simulink model "SpeedLoop"  (R2023b)
settings: Solver=FixedStepAuto  StartTime=0.0  StopTime=10.0  FixedStep=0.0001  RelTol=1e-3
values from neighbouring files (symbols this model uses):
  curr_ki = 2.3    [Speedloop.sldd]
  curr_kp = 0.0008    [Speedloop.sldd]
  Pn = 4.0    [Speedloop.sldd]
  spd_ki = 0.021    [Speedloop.sldd]
  spd_kp = 0.013    [Speedloop.sldd]
  Udc = 24.0    [Speedloop.sldd]
libraries: slpidlib x3, mcbplantlib x1, autolibpmsmexterior x1, simulink x1
settings Model: DataDictionary=Speedloop.sldd  Creator=00033411  LastModifiedBy=00033411
settings OptimizationCC: DefaultParameterBehavior=Inlined  UseDivisionForNetSlopeComputation=on  GainParamInheritBuiltInType=on  UseFloatMulNetSlope=on  InlineInvariantSignals=on  PassReuseOutputArgsAs=Individual arguments  ZeroExternalMemoryAtStartup=off  ZeroInternalMemoryAtStartup=off  NoFixptDivByZeroProtection=on  EfficientFloat2IntCast=on  LifeSpan=1  OptimizeBlockOrder=speed  DifferentSizesBufferReuse=on  EfficientTunableParamExpr=on
settings DebuggingCC: ParameterPrecisionLossMsg=none  ParameterTunabilityLossMsg=error
settings HardwareCC: ProdBitPerPointer=32  ProdBitPerSizeT=32  ProdBitPerPtrDiffT=32  ProdLargestAtomicInteger=Long  ProdLargestAtomicFloat=Double  ProdWordSize=32  ProdLongLongMode=on  ProdHWDeviceType=ARM Compatible->ARM Cortex-M
settings SFSimCC: MATLABDynamicMemAlloc=off
settings RTWCC: Description=Embedded Coder  SystemTargetFile=ert.tlc  TemplateMakefile=ert_default_tmf  GenerateReport=on  LaunchReport=on
settings CodeAppCC: ForceParamTrailComments=on  IgnoreCustomStorageClasses=off  OperatorAnnotations=on  SimulinkDataObjDesc=on  SFDataObjDesc=on  CustomSymbolStrGlobalVar=rt$N$M  CustomSymbolStrType=$N$M  CustomSymbolStrFcn=$N$M$F  CustomSymbolStrMacro=$N$M  InsertBlockDesc=on
settings ERTTargetCC: TargetLangStandard=C99 (ISO)  CodeReplacementLibrary=ARM Cortex-M  GenerateSampleERTMain=on  IncludeMdlTerminateFcn=off  CombineSignalStateStructs=on  SupportComplex=off  SupportNonInlinedSFcns=on  InlinedParameterPlacement=NonHierarchical  ERTCustomFileTemplate=example_file_process.tlc  ERTFilePackagingFormat=CompactWithDataFile

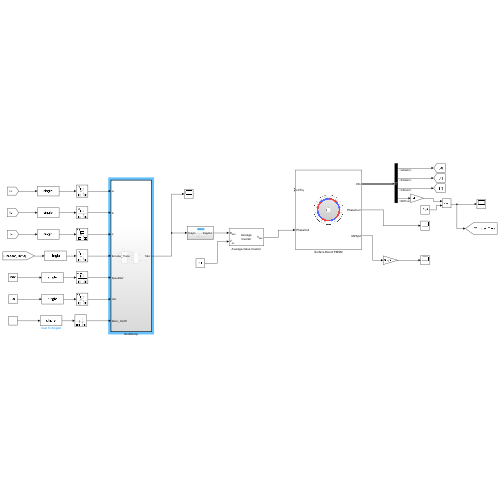
[thumbnail: Simulink's stored preview of the top-level diagram]
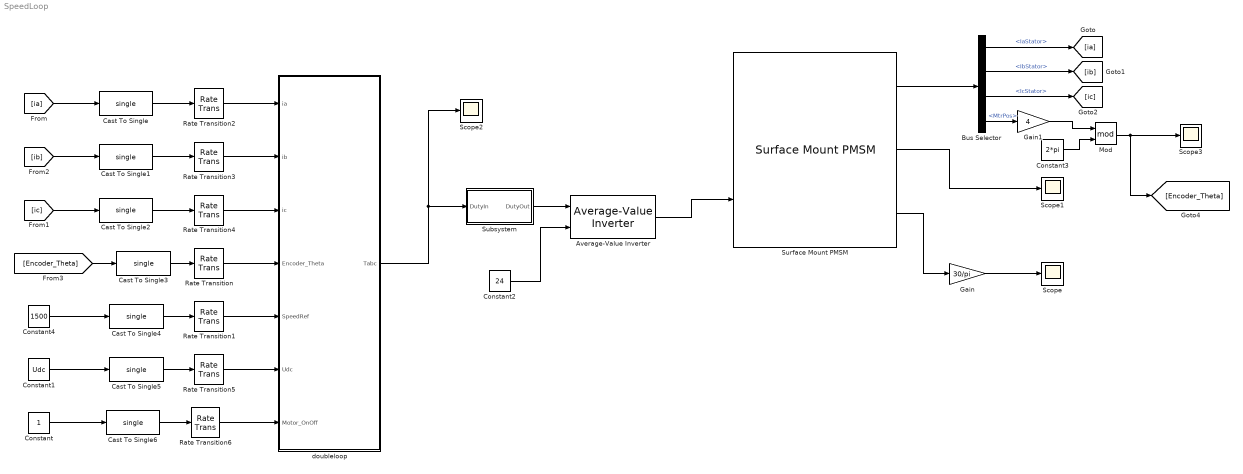
== system SpeedLoop ==
  Average-Value Inverter : mcbplantlib/Average-Value Inverter
      settings: LibrarySourceBlock=mcblib/Electrical Systems/Inverters/Average-Value Inverter
  Bus Selector : BusSelector  OutputSignals=IaStator,IbStator,IcStator,MtrPos
  Cast To Single{,1..6} (7 alike) : DataTypeConversion  OutDataTypeStr=single  SaturateOnIntegerOverflow=off  RndMeth=Floor
  Constant : Constant  OutDataTypeStr=single
  Constant1 : Constant  Value=Udc
  Constant2 : Constant  Value=24
  Constant3 : Constant  Value=2*pi
  Constant4 : Constant  Value=1500  OutDataTypeStr=single
  Gain : Gain  Gain=30/pi
  Gain1 : Gain  Gain=4
  Mod : Math  Operator=mod
  Rate Transition{,1..6} (7 alike) : RateTransition
  Scope{,1..3} (4 alike) : Scope
  Subsystem : Subsystem
  Surface Mount PMSM : autolibpmsmexterior/Surface Mount PMSM  port_config=Torque  sim_type=Discrete  Ts=1e-4  P=Pn  Rs=Rs  Ldq_=L  KConstText=Back-emf constant (Ke):  lambda_pm=3.59  Ke=Ke  Kt=1.323  mechanical=[1.55e-6, 3.86e-6, 0]  idq0=[0 0]  theta_init=0  omega_init=0  KConst=3.59  lambda_pm_calc=0.0049482  RefBlkName='autolibpmsmexterior/Surface Mount PMSM'  aMode=5  Ldq="[0.0017      0.0017]"
  doubleloop : Subsystem  TreatAsAtomicUnit=on
  wires:
  Bus Selector/1 -> [ia]  "<IaStator>"
  Bus Selector/2 -> [ib]  "<IbStator>"
  Surface Mount PMSM/2 -> Scope1/1
  Bus Selector/4 -> Gain1/1  "<MtrPos>"
  Constant3/1 -> Mod/2
  Gain/1 -> Scope/1
  Subsystem/1(DutyOut) -> Average-Value Inverter/1
  Surface Mount PMSM/3 -> Gain/1
  Constant2/1 -> Average-Value Inverter/2
  Gain1/1 -> Mod/1
  Mod/1 -> [Encoder_Theta], Scope3/1
  Average-Value Inverter/1 -> Surface Mount PMSM/2
  Bus Selector/3 -> [ic]  "<IcStator>"
  Surface Mount PMSM/1 -> Bus Selector/1
  doubleloop/1(Tabc) -> Scope2/1, Subsystem/1(DutyIn)
  Rate Transition/1 -> doubleloop/4(Encoder_Theta)
  Rate Transition6/1 -> doubleloop/7(Motor_OnOff)
  Rate Transition5/1 -> doubleloop/6(Udc)
  Rate Transition4/1 -> doubleloop/3(ic)
  Rate Transition3/1 -> doubleloop/2(ib)
  Rate Transition2/1 -> doubleloop/1(ia)
  Rate Transition1/1 -> doubleloop/5(SpeedRef)
  [ia] -> Cast To Single/1
  Cast To Single/1 -> Rate Transition2/1
  [ib] -> Cast To Single1/1
  Cast To Single1/1 -> Rate Transition3/1
  [ic] -> Cast To Single2/1
  Cast To Single2/1 -> Rate Transition4/1
  [Encoder_Theta] -> Cast To Single3/1
  Cast To Single3/1 -> Rate Transition/1
  Constant4/1 -> Cast To Single4/1
  Cast To Single4/1 -> Rate Transition1/1
  Constant1/1 -> Cast To Single5/1
  Cast To Single5/1 -> Rate Transition5/1
  Constant/1 -> Cast To Single6/1
  Cast To Single6/1 -> Rate Transition6/1

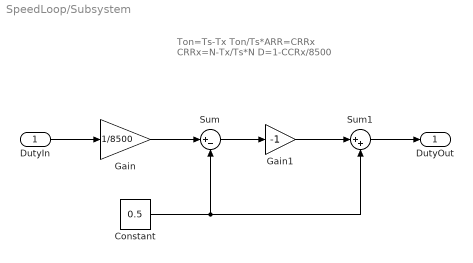
== system SpeedLoop/Subsystem ==
  note: Ton=Ts-Tx Ton/Ts*ARR=CRRx
      | CRRx=N-Tx/Ts*N
      | D=1-CCRx/8500
  DutyIn : Inport
  Constant : Constant  Value=0.5  SampleTime=-1
  Gain : Gain  Gain=1/8500  ParamDataTypeStr=single
  Gain1 : Gain  Gain=-1
  Sum : Sum  Inputs=|+-
  Sum1 : Sum  Inputs=|++
  DutyOut : Outport
  wires:
  Sum/1 -> Gain1/1
  Constant/1 -> Sum1/2, Sum/2
  DutyIn/1 -> Gain/1
  Gain1/1 -> Sum1/1
  Sum1/1 -> DutyOut/1
  Gain/1 -> Sum/1

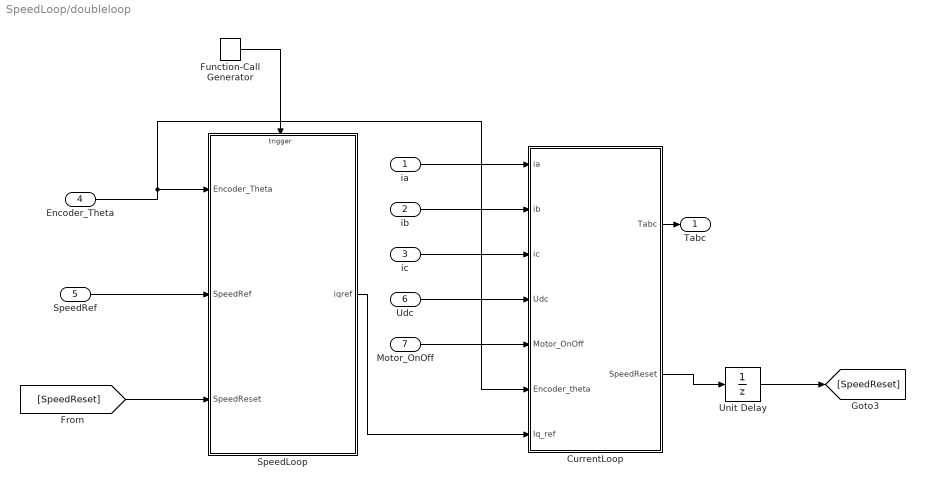
== system SpeedLoop/doubleloop ==
  ia : Inport
  ib : Inport  Port=2
  ic : Inport  Port=3
  Encoder_Theta : Inport  Port=4
  SpeedRef : Inport  Port=5
  Udc : Inport  Port=6
  Motor_OnOff : Inport  Port=7
  CurrentLoop : Subsystem
  Function-Call Generator : simulink/Ports & Subsystems/Function-Call Generator  sample_time=1e-3  numberOfIterations=1  DisallowWideOutput=off
  SpeedLoop : Subsystem  TreatAsAtomicUnit=on
  Unit Delay : UnitDelay  SampleTime=-1  HasFrameUpgradeWarning=on
  Tabc : Outport
  wires:
  [SpeedReset] -> SpeedLoop/3(SpeedReset)
  CurrentLoop/2(SpeedReset) -> Unit Delay/1
  SpeedLoop/1(iqref) -> CurrentLoop/7(Iq_ref)
  Encoder_Theta/1 -> CurrentLoop/6(Encoder_theta), SpeedLoop/1(Encoder_Theta)
  Function-Call Generator/1 -> SpeedLoop/Trigger
  Udc/1 -> CurrentLoop/4(Udc)
  Unit Delay/1 -> [SpeedReset]
  Motor_OnOff/1 -> CurrentLoop/5(Motor_OnOff)
  SpeedRef/1 -> SpeedLoop/2(SpeedRef)
  ia/1 -> CurrentLoop/1(ia)
  ic/1 -> CurrentLoop/3(ic)
  ib/1 -> CurrentLoop/2(ib)
  CurrentLoop/1(Tabc) -> Tabc/1

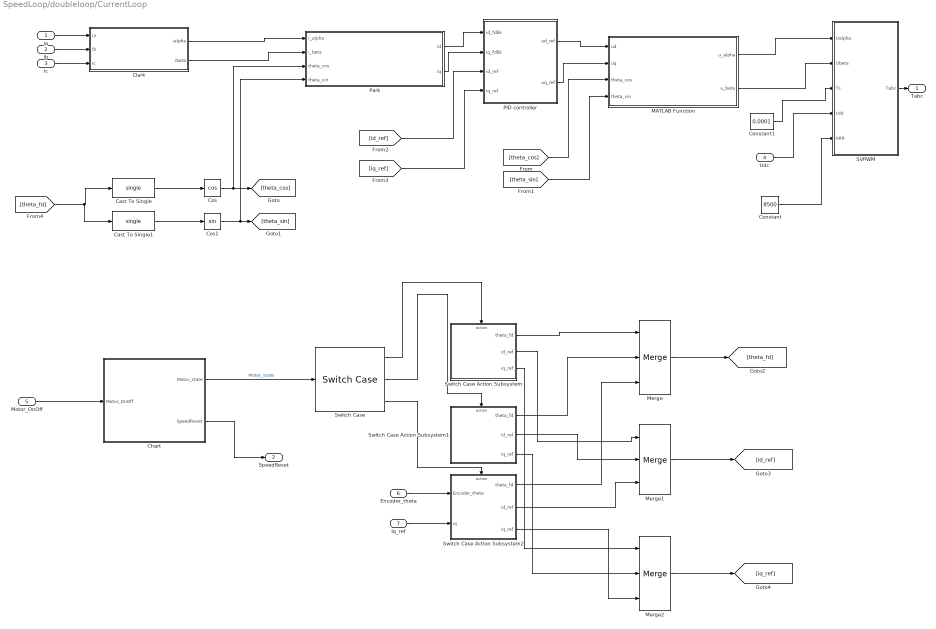
== system SpeedLoop/doubleloop/CurrentLoop ==
  ia : Inport
  ib : Inport  Port=2
  ic : Inport  Port=3
  Udc : Inport  Port=4
  Motor_OnOff : Inport  Port=5
  Encoder_theta : Inport  Port=6
  Iq_ref : Inport  Port=7
  Cast To Single : DataTypeConversion  OutDataTypeStr=single  SaturateOnIntegerOverflow=off  RndMeth=Floor
  Cast To Single1 : DataTypeConversion  OutDataTypeStr=single  SaturateOnIntegerOverflow=off  RndMeth=Floor
  Chart : Stateflow chart  TreatAsAtomicUnit=on
  Clark : MATLAB Function  TreatAsAtomicUnit=on
  Constant : Constant  Value=8500  OutDataTypeStr=single
  Constant1 : Constant  Value=0.0001  OutDataTypeStr=single
  Cos : Trigonometry  Operator=cos
  Cos1 : Trigonometry
  MATLAB Function : MATLAB Function  TreatAsAtomicUnit=on
  Merge : Merge  Inputs=3
  Merge1 : Merge  Inputs=3
  Merge2 : Merge  Inputs=3
  PID controller : Subsystem
  Park : MATLAB Function  TreatAsAtomicUnit=on
  SVPWM : Subsystem  TreatAsAtomicUnit=on
  Switch Case : SwitchCase  CaseConditions={1,2,3}  ShowDefaultCase=off
  Switch Case Action Subsystem : Subsystem  TreatAsAtomicUnit=on
  Switch Case Action Subsystem1 : Subsystem  TreatAsAtomicUnit=on
  Switch Case Action Subsystem2 : Subsystem  TreatAsAtomicUnit=on
  Tabc : Outport
  SpeedReset : Outport  Port=2
  wires:
  MATLAB Function/1(u_alpha) -> SVPWM/1(Ualpha)
  Switch Case Action Subsystem1/1(theta_fd) -> Merge/2
  Merge2/1 -> [iq_ref]
  Switch Case/1 -> Switch Case Action Subsystem/Action
  Constant1/1 -> SVPWM/3(Ts)
  [theta_sin] -> MATLAB Function/4(theta_sin)
  Switch Case Action Subsystem2/3(iq_ref) -> Merge2/3
  [theta_cos] -> MATLAB Function/3(theta_cos)
  Cast To Single/1 -> Cos/1
  MATLAB Function/2(u_beta) -> SVPWM/2(Ubeta)
  ic/1 -> Clark/3(ic)
  Chart/1(Motor_state) -> Switch Case/1  "Motor_state"
  Merge1/1 -> [id_ref]
  Park/1(id) -> PID controller/1(id_fdbk)
  [iq_ref] -> PID controller/4(iq_ref)
  PID controller/2(uq_ref) -> MATLAB Function/2(uq)
  Cos/1 -> Park/3(theta_cos), [theta_cos]
  PID controller/1(ud_ref) -> MATLAB Function/1(ud)
  Park/2(iq) -> PID controller/2(iq_fdbk)
  [theta_fd] -> Cast To Single1/1, Cast To Single/1
  Cos1/1 -> Park/4(theta_sin), [theta_sin]
  Constant/1 -> SVPWM/5(ARR)
  ia/1 -> Clark/1(ia)
  Cast To Single1/1 -> Cos1/1
  Switch Case Action Subsystem1/2(id_ref) -> Merge1/2
  Clark/1(ialpha) -> Park/1(i_alpha)
  Switch Case Action Subsystem/3(iq_ref) -> Merge2/1
  Switch Case Action Subsystem1/3(iq_ref) -> Merge2/2
  ib/1 -> Clark/2(ib)
  Udc/1 -> SVPWM/4(Udc)
  Clark/2(ibeta) -> Park/2(i_beta)
  Switch Case/2 -> Switch Case Action Subsystem1/Action
  Switch Case Action Subsystem2/2(id_ref) -> Merge1/3
  Switch Case Action Subsystem2/1(theta_fd) -> Merge/3
  Motor_OnOff/1 -> Chart/1(Motor_OnOff)
  Switch Case Action Subsystem/2(id_ref) -> Merge1/1
  Switch Case Action Subsystem/1(theta_fd) -> Merge/1
  Switch Case/3 -> Switch Case Action Subsystem2/Action
  Merge/1 -> [theta_fd]
  [id_ref] -> PID controller/3(id_ref)
  SVPWM/1(Tabc) -> Tabc/1
  Chart/2(SpeedReset) -> SpeedReset/1
  Encoder_theta/1 -> Switch Case Action Subsystem2/1(Encoder_theta)
  Iq_ref/1 -> Switch Case Action Subsystem2/2(iq)

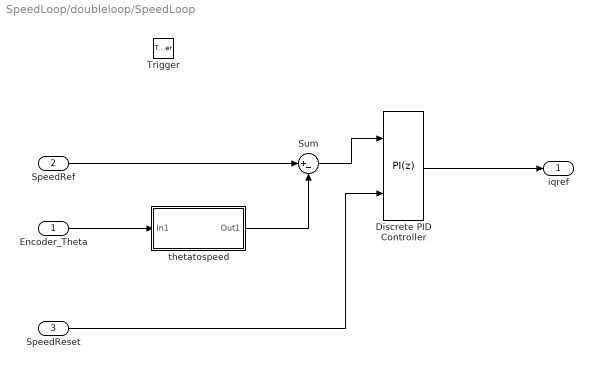
== system SpeedLoop/doubleloop/SpeedLoop ==
  Encoder_Theta : Inport
  SpeedRef : Inport  Port=2
  SpeedReset : Inport  Port=3
  Trigger : TriggerPort  TriggerType=function-call  VariantControl=(inherit)
  Discrete PID Controller : slpidlib/PID Controller  Controller=PI  Form=Parallel  TimeDomain=Discrete-time  UseExternalTs=off  SampleTime=-1  IntegratorMethod=Forward Euler  FilterMethod=Forward Euler  ControllerParametersSource=internal  P=spd_kp  I=spd_ki  UseKiTs=off  D=0  N=100  UseFilter=on  TunerSelectOption=Transfer Function Based (PID Tuner App)  InitialConditionSource=internal  InitialConditionForIntegrator=0  InitialConditionForFilter=0  DifferentiatorICPrevScaledInput=0  ExternalReset=rising  TrackingMode=off  Kt=1  LimitOutput=on  SatLimitsSource=internal  UpperSaturationLimit=20  LowerSaturationLimit=-20  LinearizeAsGain=on  AntiWindupMode=clamping  Kb=1  LimitIntegrator=off  UpperIntegratorSaturationLimit=inf  LowerIntegratorSaturationLimit=-inf  POutMin=[]  POutMax=[]  IOutMin=[]  IOutMax=[]  DOutMin=[]  DOutMax=[]  NOutMin=[]  NOutMax=[]  SumOutMin=[]  SumOutMax=[]  SaturationOutMin=[]  SaturationOutMax=[]  PParamMin=[]  PParamMax=[]  IParamMin=[]  IParamMax=[]  DParamMin=[]  DParamMax=[]  NParamMin=[]  NParamMax=[]  KbParamMin=[]  KbParamMax=[]  KtParamMin=[]  KtParamMax=[]  KbOutMin=[]  KbOutMax=[]  KtOutMin=[]  KtOutMax=[]  IntegratorOutMin=[]  IntegratorOutMax=[]  FilterOutMin=[]  FilterOutMax=[]  SumI1OutMin=[]  SumI1OutMax=[]  SumI2OutMin=[]  SumI2OutMax=[]  SumI3OutMin=[]  SumI3OutMax=[]  SumI4OutMin=[]  SumI4OutMax=[]  SumDOutMin=[]  SumDOutMax=[]  DifferentiatorOutMin=[]  DifferentiatorOutMax=[]  FilterDiffOutCoefMin=[]  FilterDiffOutCoefMax=[]  ReciprocalOutMin=[]  ReciprocalOutMax=[]  SumDenOutMin=[]  SumDenOutMax=[]  SumNumOutMin=[]  SumNumOutMax=[]  DivideOutMin=[]  DivideOutMax=[]  UdiffTsProdOutMin=[]  UdiffTsProdOutMax=[]  NTsProdOutMin=[]  NTsProdOutMax=[]  UintegralTsProdOutMin=[]  UintegralTsProdOutMax=[]  UngainTsProdOutMin=[]  UngainTsProdOutMax=[]  ClampingZeroOutDataTypeStr=Inherit: Inherit via back propagation  ClampingZeroOutMin=[]  ClampingZeroOutMax=[]  FilterDenConstantOutDataTypeStr=Inherit: Inherit via back propagation  FilterDenConstantOutMin=[]  FilterDenConstantOutMax=[]  PCopyOutDataTypeStr=Inherit: Inherit via back propagation  PCopyOutMin=[]  PCopyOutMax=[]  NCopyOutDataTypeStr=Inherit: Inherit via back propagation  NCopyOutMin=[]  NCopyOutMax=[]  IntegratorContinuousStateAttributes=''  IntegratorStateMustResolveToSignalObject=off  IntegratorRTWStateStorageClass=Auto  FilterContinuousStateAttributes=''  FilterStateMustResolveToSignalObject=off  FilterRTWStateStorageClass=Auto  ParallelPVariant=InternalParameters  IdealPVariant=Disabled  IVariant=InternalParameters  DVariant=Disabled  IntegratorVariant=Discrete  SatVariant=Enabled  AWVariant=DiscClampingParallel  PCopyVariant=Disabled  TRVariant=Disabled  FdbkBlocksVariant=Forward  IdealPFdbkVariant=Disabled  SatFdbkVariant=Disabled  DerivativeFilterVariant=Disabled  NVariant=Disabled  NCopyVariant=Disabled_SignalSpec  FilterICVariant=Disabled  IntegratorICVariant=InternalICs  ExternalResetVariant=ExternalReset  TRSumVariant=Passthrough  SumFdbkVariant=Disabled  SumVariant=Sum_PI  TsampFilterVariant=InternalTs  TsampNgainVariant=Passthrough  TsampIntegralVariant=Disabled_SignalSpec  ExternalSaturationOutDataTypeStr=Inherit: Same as second input
      settings: LibrarySourceBlock=simulink/Discrete/Discrete PID Controller
  Sum : Sum  Inputs=|+-
  thetatospeed : Subsystem
  iqref : Outport
  wires:
  Encoder_Theta/1 -> thetatospeed/1(In1)
  SpeedRef/1 -> Sum/1
  thetatospeed/1(Out1) -> Sum/2
  Sum/1 -> Discrete PID Controller/1
  SpeedReset/1 -> Discrete PID Controller/2
  Discrete PID Controller/1 -> iqref/1

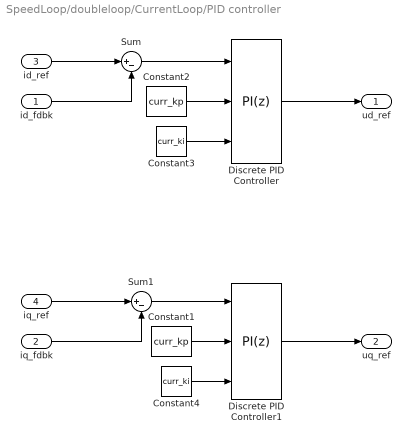
== system SpeedLoop/doubleloop/CurrentLoop/PID controller ==
  id_fdbk : Inport
  iq_fdbk : Inport  Port=2
  id_ref : Inport  Port=3
  iq_ref : Inport  Port=4
  Constant1 : Constant  Value=curr_kp
  Constant2 : Constant  Value=curr_kp
  Constant3 : Constant  Value=curr_ki
  Constant4 : Constant  Value=curr_ki
  Discrete PID Controller : slpidlib/PID Controller  Controller=PI  Form=Parallel  TimeDomain=Discrete-time  UseExternalTs=off  SampleTime=-1  IntegratorMethod=Forward Euler  FilterMethod=Forward Euler  ControllerParametersSource=external  P=1  I=1  UseKiTs=off  D=0  N=100  UseFilter=on  TunerSelectOption=Transfer Function Based (PID Tuner App)  InitialConditionSource=internal  InitialConditionForIntegrator=0  InitialConditionForFilter=0  DifferentiatorICPrevScaledInput=0  ExternalReset=none  TrackingMode=off  Kt=1  LimitOutput=off  SatLimitsSource=internal  UpperSaturationLimit=24*0.9/sqrt(3)  LowerSaturationLimit=-24*0.9/sqrt(3)  LinearizeAsGain=off  AntiWindupMode=clamping  Kb=1  LimitIntegrator=off  UpperIntegratorSaturationLimit=inf  LowerIntegratorSaturationLimit=-inf  POutMin=[]  POutMax=[]  IOutMin=[]  IOutMax=[]  DOutMin=[]  DOutMax=[]  NOutMin=[]  NOutMax=[]  SumOutMin=[]  SumOutMax=[]  SaturationOutMin=[]  SaturationOutMax=[]  PParamMin=[]  PParamMax=[]  IParamMin=[]  IParamMax=[]  DParamMin=[]  DParamMax=[]  NParamMin=[]  NParamMax=[]  KbParamMin=[]  KbParamMax=[]  KtParamMin=[]  KtParamMax=[]  KbOutMin=[]  KbOutMax=[]  KtOutMin=[]  KtOutMax=[]  IntegratorOutMin=[]  IntegratorOutMax=[]  FilterOutMin=[]  FilterOutMax=[]  SumI1OutMin=[]  SumI1OutMax=[]  SumI2OutMin=[]  SumI2OutMax=[]  SumI3OutMin=[]  SumI3OutMax=[]  SumI4OutMin=[]  SumI4OutMax=[]  SumDOutMin=[]  SumDOutMax=[]  DifferentiatorOutMin=[]  DifferentiatorOutMax=[]  FilterDiffOutCoefMin=[]  FilterDiffOutCoefMax=[]  ReciprocalOutMin=[]  ReciprocalOutMax=[]  SumDenOutMin=[]  SumDenOutMax=[]  SumNumOutMin=[]  SumNumOutMax=[]  DivideOutMin=[]  DivideOutMax=[]  UdiffTsProdOutMin=[]  UdiffTsProdOutMax=[]  NTsProdOutMin=[]  NTsProdOutMax=[]  UintegralTsProdOutMin=[]  UintegralTsProdOutMax=[]  UngainTsProdOutMin=[]  UngainTsProdOutMax=[]  ClampingZeroOutDataTypeStr=Inherit: Inherit via back propagation  ClampingZeroOutMin=[]  ClampingZeroOutMax=[]  FilterDenConstantOutDataTypeStr=Inherit: Inherit via back propagation  FilterDenConstantOutMin=[]  FilterDenConstantOutMax=[]  PCopyOutDataTypeStr=Inherit: Inherit via back propagation  PCopyOutMin=[]  PCopyOutMax=[]  NCopyOutDataTypeStr=Inherit: Inherit via back propagation  NCopyOutMin=[]  NCopyOutMax=[]  IntegratorContinuousStateAttributes=''  IntegratorStateMustResolveToSignalObject=off  IntegratorRTWStateStorageClass=Auto  FilterContinuousStateAttributes=''  FilterStateMustResolveToSignalObject=off  FilterRTWStateStorageClass=Auto  ParallelPVariant=ExternalParameters  IdealPVariant=Disabled  IVariant=ExternalParameters  DVariant=Disabled  IntegratorVariant=Discrete  SatVariant=Disabled  AWVariant=Passthrough  PCopyVariant=Disabled  TRVariant=Disabled  FdbkBlocksVariant=Forward  IdealPFdbkVariant=Disabled  SatFdbkVariant=Disabled  DerivativeFilterVariant=Disabled  NVariant=Disabled  NCopyVariant=Disabled_SignalSpec  FilterICVariant=Disabled  IntegratorICVariant=InternalICs  ExternalResetVariant=Disabled  TRSumVariant=Passthrough  SumFdbkVariant=Disabled  SumVariant=Sum_PI  TsampFilterVariant=InternalTs  TsampNgainVariant=Passthrough  TsampIntegralVariant=Disabled_SignalSpec  ExternalSaturationOutDataTypeStr=Inherit: Same as second input
      settings: LibrarySourceBlock=simulink/Discrete/Discrete PID Controller
  Discrete PID Controller1 : slpidlib/PID Controller  Controller=PI  Form=Parallel  TimeDomain=Discrete-time  UseExternalTs=off  SampleTime=-1  IntegratorMethod=Forward Euler  FilterMethod=Forward Euler  ControllerParametersSource=external  P=1  I=1  UseKiTs=off  D=0  N=100  UseFilter=on  TunerSelectOption=Transfer Function Based (PID Tuner App)  InitialConditionSource=internal  InitialConditionForIntegrator=0  InitialConditionForFilter=0  DifferentiatorICPrevScaledInput=0  ExternalReset=none  TrackingMode=off  Kt=1  LimitOutput=on  SatLimitsSource=internal  UpperSaturationLimit=24*0.9/sqrt(3)  LowerSaturationLimit=-24*0.9/sqrt(3)  LinearizeAsGain=on  AntiWindupMode=clamping  Kb=1  LimitIntegrator=off  UpperIntegratorSaturationLimit=inf  LowerIntegratorSaturationLimit=-inf  POutMin=[]  POutMax=[]  IOutMin=[]  IOutMax=[]  DOutMin=[]  DOutMax=[]  NOutMin=[]  NOutMax=[]  SumOutMin=[]  SumOutMax=[]  SaturationOutMin=[]  SaturationOutMax=[]  PParamMin=[]  PParamMax=[]  IParamMin=[]  IParamMax=[]  DParamMin=[]  DParamMax=[]  NParamMin=[]  NParamMax=[]  KbParamMin=[]  KbParamMax=[]  KtParamMin=[]  KtParamMax=[]  KbOutMin=[]  KbOutMax=[]  KtOutMin=[]  KtOutMax=[]  IntegratorOutMin=[]  IntegratorOutMax=[]  FilterOutMin=[]  FilterOutMax=[]  SumI1OutMin=[]  SumI1OutMax=[]  SumI2OutMin=[]  SumI2OutMax=[]  SumI3OutMin=[]  SumI3OutMax=[]  SumI4OutMin=[]  SumI4OutMax=[]  SumDOutMin=[]  SumDOutMax=[]  DifferentiatorOutMin=[]  DifferentiatorOutMax=[]  FilterDiffOutCoefMin=[]  FilterDiffOutCoefMax=[]  ReciprocalOutMin=[]  ReciprocalOutMax=[]  SumDenOutMin=[]  SumDenOutMax=[]  SumNumOutMin=[]  SumNumOutMax=[]  DivideOutMin=[]  DivideOutMax=[]  UdiffTsProdOutMin=[]  UdiffTsProdOutMax=[]  NTsProdOutMin=[]  NTsProdOutMax=[]  UintegralTsProdOutMin=[]  UintegralTsProdOutMax=[]  UngainTsProdOutMin=[]  UngainTsProdOutMax=[]  ClampingZeroOutDataTypeStr=Inherit: Inherit via back propagation  ClampingZeroOutMin=[]  ClampingZeroOutMax=[]  FilterDenConstantOutDataTypeStr=Inherit: Inherit via back propagation  FilterDenConstantOutMin=[]  FilterDenConstantOutMax=[]  PCopyOutDataTypeStr=Inherit: Inherit via back propagation  PCopyOutMin=[]  PCopyOutMax=[]  NCopyOutDataTypeStr=Inherit: Inherit via back propagation  NCopyOutMin=[]  NCopyOutMax=[]  IntegratorContinuousStateAttributes=''  IntegratorStateMustResolveToSignalObject=off  IntegratorRTWStateStorageClass=Auto  FilterContinuousStateAttributes=''  FilterStateMustResolveToSignalObject=off  FilterRTWStateStorageClass=Auto  ParallelPVariant=ExternalParameters  IdealPVariant=Disabled  IVariant=ExternalParameters  DVariant=Disabled  IntegratorVariant=Discrete  SatVariant=Enabled  AWVariant=DiscClampingParallel  PCopyVariant=Disabled  TRVariant=Disabled  FdbkBlocksVariant=Forward  IdealPFdbkVariant=Disabled  SatFdbkVariant=Disabled  DerivativeFilterVariant=Disabled  NVariant=Disabled  NCopyVariant=Disabled_SignalSpec  FilterICVariant=Disabled  IntegratorICVariant=InternalICs  ExternalResetVariant=Disabled  TRSumVariant=Passthrough  SumFdbkVariant=Disabled  SumVariant=Sum_PI  TsampFilterVariant=InternalTs  TsampNgainVariant=Passthrough  TsampIntegralVariant=Disabled_SignalSpec  ExternalSaturationOutDataTypeStr=Inherit: Same as second input
      settings: LibrarySourceBlock=simulink/Discrete/Discrete PID Controller
  Sum : Sum  Inputs=|+-
  Sum1 : Sum  Inputs=|+-
  ud_ref : Outport
  uq_ref : Outport  Port=2
  wires:
  Sum1/1 -> Discrete PID Controller1/1
  Sum/1 -> Discrete PID Controller/1
  Discrete PID Controller1/1 -> uq_ref/1
  Discrete PID Controller/1 -> ud_ref/1
  id_ref/1 -> Sum/1
  id_fdbk/1 -> Sum/2
  iq_ref/1 -> Sum1/1
  iq_fdbk/1 -> Sum1/2
  Constant2/1 -> Discrete PID Controller/2
  Constant3/1 -> Discrete PID Controller/3
  Constant1/1 -> Discrete PID Controller1/2
  Constant4/1 -> Discrete PID Controller1/3

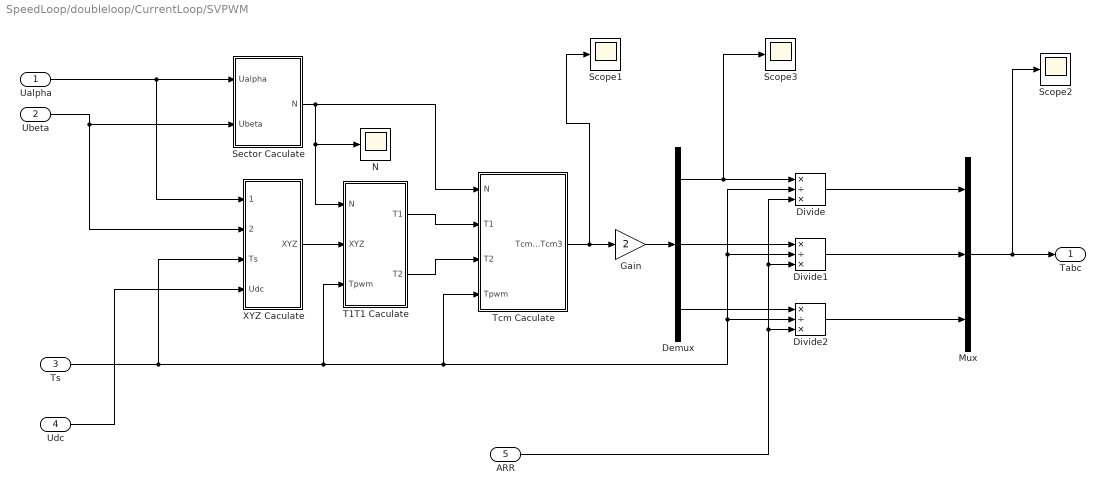
== system SpeedLoop/doubleloop/CurrentLoop/SVPWM ==
  Ualpha : Inport
  Ubeta : Inport  Port=2
  Ts : Inport  Port=3
  Udc : Inport  Port=4
  ARR : Inport  Port=5
  Demux : Demux  Outputs=3
  Divide : Product  Inputs=*/*
  Divide1 : Product  Inputs=*/*
  Divide2 : Product  Inputs=*/*
  Gain : Gain  Gain=2
  Mux : Mux  Inputs=3
  N : Scope
  Scope1 : Scope
  Scope2 : Scope
  Scope3 : Scope
  Sector Caculate : Subsystem
  T1T1 Caculate : Subsystem
  Tcm Caculate : Subsystem
  XYZ Caculate : Subsystem
  Tabc : Outport
  wires:
  Tcm Caculate/1(Tcm1 Tcm2 Tcm3) -> Gain/1, Scope1/1
  Divide1/1 -> Mux/2
  T1T1 Caculate/1(T1) -> Tcm Caculate/2(T1)
  Divide/1 -> Mux/1
  ARR/1 -> Divide2/3, Divide1/3, Divide/3
  Sector Caculate/1("N ") -> Tcm Caculate/1(N), N/1, T1T1 Caculate/1(N)
  T1T1 Caculate/2(T2) -> Tcm Caculate/3(T2)
  Ubeta/1 -> XYZ Caculate/2(Ubeta), Sector Caculate/2(Ubeta)
  Ualpha/1 -> XYZ Caculate/1(Ualpha), Sector Caculate/1(Ualpha)
  XYZ Caculate/1(XYZ) -> T1T1 Caculate/2(XYZ)
  Gain/1 -> Demux/1
  Mux/1 -> Scope2/1, Tabc/1
  Divide2/1 -> Mux/3
  Demux/1 -> Scope3/1, Divide/1
  Demux/3 -> Divide2/1
  Demux/2 -> Divide1/1
  Ts/1 -> Divide2/2, Divide1/2, Divide/2, Tcm Caculate/4(Tpwm), T1T1 Caculate/3(Tpwm), XYZ Caculate/3(Ts)
  Udc/1 -> XYZ Caculate/4(Udc)

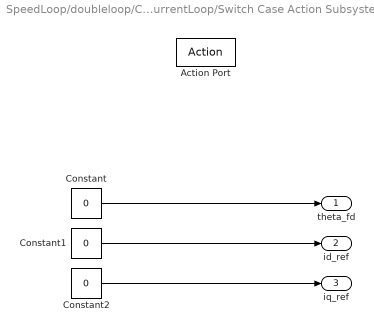
== system SpeedLoop/doubleloop/CurrentLoop/Switch Case Action Subsystem ==
  Action Port : ActionPort  ActionPortLabel=case [ 1 ]:
  Constant : Constant  Value=0  OutDataTypeStr=single
  Constant1 : Constant  Value=0  OutDataTypeStr=single
  Constant2 : Constant  Value=0  OutDataTypeStr=single
  theta_fd : Outport
  id_ref : Outport  Port=2
  iq_ref : Outport  Port=3
  wires:
  Constant/1 -> theta_fd/1
  Constant1/1 -> id_ref/1
  Constant2/1 -> iq_ref/1

== system SpeedLoop/doubleloop/CurrentLoop/Switch Case Action Subsystem1 ==
  Action Port : ActionPort  ActionPortLabel=case [ 2 ]:
  Constant : Constant  Value=0  OutDataTypeStr=single
  Constant1 : Constant  Value=2  OutDataTypeStr=single
  Constant2 : Constant  Value=0  OutDataTypeStr=single
  theta_fd : Outport
  id_ref : Outport  Port=2
  iq_ref : Outport  Port=3
  wires:
  Constant/1 -> theta_fd/1
  Constant1/1 -> id_ref/1
  Constant2/1 -> iq_ref/1

== system SpeedLoop/doubleloop/CurrentLoop/Switch Case Action Subsystem2 ==
  Encoder_theta : Inport
  iq : Inport  Port=2
  Action Port : ActionPort  ActionPortLabel=case [ 3 ]:
  Constant1 : Constant  Value=0  OutDataTypeStr=single
  theta_fd : Outport
  id_ref : Outport  Port=2
  iq_ref : Outport  Port=3
  wires:
  iq/1 -> iq_ref/1
  Constant1/1 -> id_ref/1
  Encoder_theta/1 -> theta_fd/1

== system SpeedLoop/doubleloop/SpeedLoop/thetatospeed ==
  In1 : Inport
  AngleLimit : Subsystem
  Gain : Gain  Gain=30/pi
  Gain1 : Gain  Gain=1/4
  Sum : Sum  Inputs=|+-
  Unit Delay : UnitDelay  SampleTime=-1  HasFrameUpgradeWarning=on
  Out1 : Outport
  wires:
  Unit Delay/1 -> Sum/2
  In1/1 -> Unit Delay/1, Sum/1
  Sum/1 -> AngleLimit/1(In1)
  Gain/1 -> Gain1/1
  AngleLimit/1(Out1) -> Gain/1
  Gain1/1 -> Out1/1  "SpeedFd"

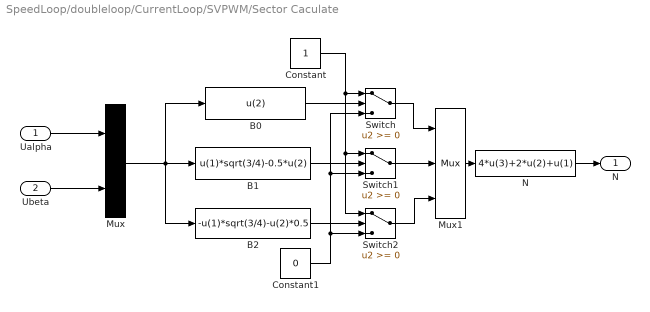
== system SpeedLoop/doubleloop/CurrentLoop/SVPWM/Sector Caculate ==
  Ualpha : Inport
  Ubeta : Inport  Port=2
  B0 : Fcn  Expr=u(2)
  B1 : Fcn  Expr=u(1)*sqrt(3/4)-0.5*u(2)
  B2 : Fcn  Expr=-u(1)*sqrt(3/4)-u(2)*0.5
  Constant : Constant
  Constant1 : Constant  Value=0
  Mux : Mux  Inputs=2
  Mux1 : Mux  Inputs=3
  N : Fcn  Expr=4*u(3)+2*u(2)+u(1)
  Switch : Switch  SaturateOnIntegerOverflow=off  InputSameDT=off
  Switch1 : Switch  SaturateOnIntegerOverflow=off  InputSameDT=off
  Switch2 : Switch  SaturateOnIntegerOverflow=off  InputSameDT=off
  "N " : Outport
  wires:
  Switch2/1 -> Mux1/3
  Switch/1 -> Mux1/1
  Ualpha/1 -> Mux/1
  Ubeta/1 -> Mux/2
  Mux/1 -> B2/1, B1/1, B0/1
  B0/1 -> Switch/2
  B1/1 -> Switch1/2
  B2/1 -> Switch2/2
  Constant/1 -> Switch/1, Switch2/1, Switch1/1
  Constant1/1 -> Switch/3, Switch1/3, Switch2/3
  Switch1/1 -> Mux1/2
  Mux1/1 -> N/1
  N/1 -> "N "/1

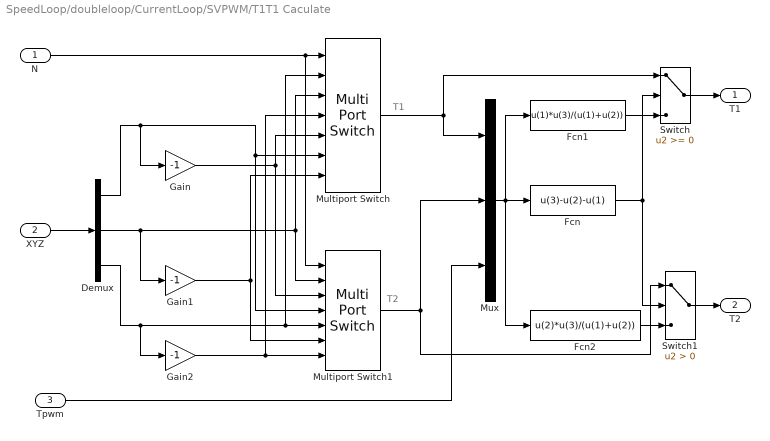
== system SpeedLoop/doubleloop/CurrentLoop/SVPWM/T1T1 Caculate ==
  note: T1
  note: T2
  N : Inport
  XYZ : Inport  Port=2
  Tpwm : Inport  Port=3
  Demux : Demux  Outputs=3
  Fcn : Fcn  Expr=u(3)-u(2)-u(1)
  Fcn1 : Fcn  Expr=u(1)*u(3)/(u(1)+u(2))
  Fcn2 : Fcn  Expr=u(2)*u(3)/(u(1)+u(2))
  Gain : Gain  Gain=-1
  Gain1 : Gain  Gain=-1
  Gain2 : Gain  Gain=-1
  Multiport Switch : MultiPortSwitch  Inputs=6  DiagnosticForDefault=None  SaturateOnIntegerOverflow=off  InputSameDT=off
  Multiport Switch1 : MultiPortSwitch  Inputs=6  DiagnosticForDefault=None  SaturateOnIntegerOverflow=off  InputSameDT=off
  Mux : Mux  Inputs=3
  Switch : Switch  SaturateOnIntegerOverflow=off  InputSameDT=off
  Switch1 : Switch  Criteria=u2 > Threshold  SaturateOnIntegerOverflow=off  InputSameDT=off
  T1 : Outport
  T2 : Outport  Port=2
  wires:
  Tpwm/1 -> Mux/3
  XYZ/1 -> Demux/1
  Switch1/1 -> T2/1
  Switch/1 -> T1/1
  Fcn2/1 -> Switch1/3
  Fcn1/1 -> Switch/3
  Fcn/1 -> Switch/2, Switch1/2
  Mux/1 -> Fcn1/1, Fcn/1, Fcn2/1
  Multiport Switch/1 -> Switch/1, Mux/1
  Multiport Switch1/1 -> Switch1/1, Mux/2
  N/1 -> Multiport Switch/1, Multiport Switch1/1
  Demux/2 -> Multiport Switch/3, Multiport Switch1/2, Gain1/1
  Demux/3 -> Multiport Switch1/5, Multiport Switch/2, Gain2/1
  Demux/1 -> Multiport Switch/6, Multiport Switch1/4, Gain/1
  Gain/1 -> Multiport Switch1/3, Multiport Switch/5
  Gain2/1 -> Multiport Switch/4, Multiport Switch1/7
  Gain1/1 -> Multiport Switch1/6, Multiport Switch/7

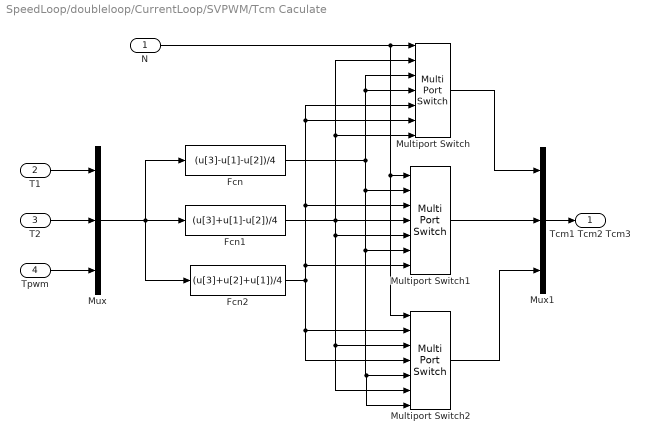
== system SpeedLoop/doubleloop/CurrentLoop/SVPWM/Tcm Caculate ==
  N : Inport
  T1 : Inport  Port=2
  T2 : Inport  Port=3
  Tpwm : Inport  Port=4
  Fcn : Fcn  Expr=(u[3]-u[1]-u[2])/4
  Fcn1 : Fcn  Expr=(u[3]+u[1]-u[2])/4
  Fcn2 : Fcn  Expr=(u[3]+u[2]+u[1])/4
  Multiport Switch : MultiPortSwitch  Inputs=6  DiagnosticForDefault=None  SaturateOnIntegerOverflow=off  InputSameDT=off
  Multiport Switch1 : MultiPortSwitch  Inputs=6  DiagnosticForDefault=None  SaturateOnIntegerOverflow=off  InputSameDT=off
  Multiport Switch2 : MultiPortSwitch  Inputs=6  DiagnosticForDefault=None  SaturateOnIntegerOverflow=off  InputSameDT=off
  Mux : Mux  Inputs=3
  Mux1 : Mux  Inputs=3
  Tcm1 Tcm2 Tcm3 : Outport
  wires:
  Mux/1 -> Fcn2/1, Fcn/1, Fcn1/1
  Tpwm/1 -> Mux/3
  T2/1 -> Mux/2
  T1/1 -> Mux/1
  Multiport Switch2/1 -> Mux1/3
  Multiport Switch1/1 -> Mux1/2
  Multiport Switch/1 -> Mux1/1
  Mux1/1 -> Tcm1 Tcm2 Tcm3/1
  Fcn/1 -> Multiport Switch/3, Multiport Switch/4, Multiport Switch1/6, Multiport Switch2/5, Multiport Switch2/7, Multiport Switch1/2
  Fcn1/1 -> Multiport Switch1/5, Multiport Switch2/3, Multiport Switch2/6, Multiport Switch1/4, Multiport Switch/7, Multiport Switch/2
  Fcn2/1 -> Multiport Switch/5, Multiport Switch/6, Multiport Switch1/3, Multiport Switch1/7, Multiport Switch2/2, Multiport Switch2/4
  N/1 -> Multiport Switch2/1, Multiport Switch1/1, Multiport Switch/1

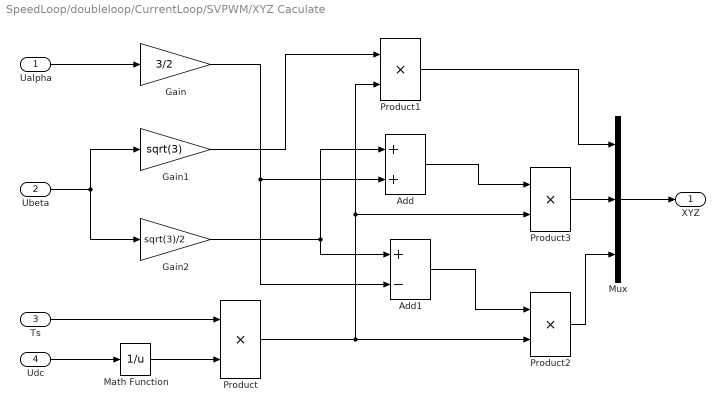
== system SpeedLoop/doubleloop/CurrentLoop/SVPWM/XYZ Caculate ==
  Ualpha : Inport
  Ubeta : Inport  Port=2
  Ts : Inport  Port=3
  Udc : Inport  Port=4
  Add : Sum
  Add1 : Sum  Inputs=+-
  Gain : Gain  Gain=3/2
  Gain1 : Gain  Gain=sqrt(3)
  Gain2 : Gain  Gain=sqrt(3)/2
  Math Function : Math  Operator=reciprocal  SignedPower=on
  Mux : Mux  Inputs=3
  Product{,1..3} (4 alike) : Product  RndMeth=Zero
  XYZ : Outport
  wires:
  Mux/1 -> XYZ/1
  Product1/1 -> Mux/1
  Product3/1 -> Mux/2
  Product2/1 -> Mux/3
  Ualpha/1 -> Gain/1
  Ubeta/1 -> Gain2/1, Gain1/1
  Udc/1 -> Math Function/1
  Math Function/1 -> Product/2
  Ts/1 -> Product/1
  Gain1/1 -> Product1/1
  Product/1 -> Product2/2, Product1/2, Product3/2
  Gain/1 -> Add1/2, Add/2
  Gain2/1 -> Add/1, Add1/1
  Add1/1 -> Product2/1
  Add/1 -> Product3/1

== system SpeedLoop/doubleloop/SpeedLoop/thetatospeed/AngleLimit ==
  In1 : Inport
  If : If  IfExpression=u1 > single(4.2)  ElseIfExpressions=u1 < single(-4.2)
  If Action Subsystem : Subsystem  TreatAsAtomicUnit=on
  If Action Subsystem1 : Subsystem  TreatAsAtomicUnit=on
  If Action Subsystem2 : Subsystem  TreatAsAtomicUnit=on
  Merge : Merge  Inputs=3
  Out1 : Outport
  wires:
  In1/1 -> If Action Subsystem1/1(In1), If Action Subsystem2/1(In1), If Action Subsystem/1(In1), If/1
  If/1 -> If Action Subsystem/Action
  If/2 -> If Action Subsystem1/Action
  If/3 -> If Action Subsystem2/Action
  If Action Subsystem/1(Out1) -> Merge/1
  If Action Subsystem1/1(Out1) -> Merge/2
  If Action Subsystem2/1(Out1) -> Merge/3
  Merge/1 -> Out1/1

== system SpeedLoop/doubleloop/SpeedLoop/thetatospeed/AngleLimit/If Action Subsystem ==
  In1 : Inport
  Action Port : ActionPort  ActionPortLabel=if(u1 > single(4.2))
  Constant : Constant  Value=2*pi  OutDataTypeStr=single
  Gain : Gain  Gain=1000
  Subtract : Sum  Inputs=+-
  Out1 : Outport
  wires:
  In1/1 -> Subtract/1
  Constant/1 -> Subtract/2
  Subtract/1 -> Gain/1
  Gain/1 -> Out1/1

== system SpeedLoop/doubleloop/SpeedLoop/thetatospeed/AngleLimit/If Action Subsystem1 ==
  In1 : Inport
  Action Port : ActionPort  ActionPortLabel=elseif(u1 < single(-4.2))
  Constant : Constant  Value=2*pi  OutDataTypeStr=single
  Gain : Gain  Gain=1000
  Subtract : Sum
  Out1 : Outport
  wires:
  In1/1 -> Subtract/1
  Constant/1 -> Subtract/2
  Subtract/1 -> Gain/1
  Gain/1 -> Out1/1

== system SpeedLoop/doubleloop/SpeedLoop/thetatospeed/AngleLimit/If Action Subsystem2 ==
  In1 : Inport
  Action Port : ActionPort  ActionPortLabel=else
  Gain : Gain  Gain=1000
  Out1 : Outport
  wires:
  In1/1 -> Gain/1
  Gain/1 -> Out1/1

== matlab function SpeedLoop/doubleloop/CurrentLoop/Park ==
  data: i_alpha input; id output; i_beta input; theta_cos input; theta_sin input; iq output
function [id, iq] = Park(i_alpha, i_beta, theta_cos, theta_sin)
% ==============================
% 标准Park变换 (αβ静止坐标系 → dq旋转坐标系)
% 输入：不使用theta！直接用预计算的 cosθ 和 sinθ
% i_alpha   : α轴电流
% i_beta    : β轴电流
% theta_cos : 电角度余弦值 cos(θ)
% theta_sin : 电角度正弦值 sin(θ)
% 输出：
% id : d轴励磁电流
% iq : q轴转矩电流
% ==============================

% 标准Park公式（直接代入cosθ/sinθ，无三角函数运算）
id = i_alpha * theta_cos + i_beta * theta_sin;
iq = -i_alpha * theta_sin + i_beta * theta_cos;
end

== matlab function SpeedLoop/doubleloop/CurrentLoop/Clark ==
  data: ia input; ialpha output; ib input; ic input; ibeta output
function [ialpha, ibeta] = clark_current_equal_amp(ia, ib, ic)
% 电流等幅值Clark变换 (三相静止abc → 两相静止αβ)
% 输入：ia, ib, ic - 三相瞬时电流
% 输出：ialpha, ibeta - αβ轴电流分量

sqrt3 = sqrt(3); % 定义√3常数

% 等幅值变换核心公式
ialpha = (2*ia - ib - ic) / 3;  
ibeta  = sqrt3 * (ib - ic) / 3;  
end

== stateflow chart SpeedLoop/doubleloop/CurrentLoop/Chart ==
  state IDLE
    en:
    du:
    Motor_state=1;
  state AlignStage
    en:
    SpeedReset=0;
    du:
    Motor_state=2;
  state RunStage
    en:
    SpeedReset=1;
    du:
    Motor_state=3;
  (default) -> IDLE
  IDLE -> AlignStage : [Motor_OnOff==1]
  AlignStage -> RunStage [order 1] : after(2000,tick)
  RunStage -> IDLE : [Motor_OnOff==0]
  AlignStage -> IDLE [order 2] : [Motor_OnOff==0]
  data: Motor_state output single; Motor_OnOff input single; SpeedReset output single

== matlab function SpeedLoop/doubleloop/CurrentLoop/MATLAB Function ==
  data: ud input; u_alpha output; uq input; theta_cos input; theta_sin input; u_beta output
function [u_alpha, u_beta] = InvPark(ud, uq, theta_cos, theta_sin)
% ==============================
% 标准反Park变换 (dq旋转坐标系 → αβ静止坐标系)
% 输入：不使用theta！直接用预计算的 cosθ 和 sinθ
% ud        : d轴电压
% uq        : q轴电压
% theta_cos : 电角度余弦值 cos(θ)
% theta_sin : 电角度正弦值 sin(θ)
% 输出：
% u_alpha : α轴电压
% u_beta  : β轴电压
% ==============================

% 标准反Park公式（直接代入cosθ/sinθ，无三角函数运算）
u_alpha = ud * theta_cos - uq * theta_sin;
u_beta  = ud * theta_sin + uq * theta_cos;
end
